simulink model "CritLike"  (R2018a)
settings: Solver=VariableStepAuto  StartTime=0.0  StopTime=0.001  RelTol=1e-3
undefined symbols (not defined in the file or in its folder): fdesignblkfcn, G1, G2, G3, G4, G5, G6, G7, G8, gcbh, get, T
libraries: dspsrcs4 x1, dspxfrm3 x1, dspobslib x1
settings Model: Creator=Daniel  LastModifiedBy=Daniel

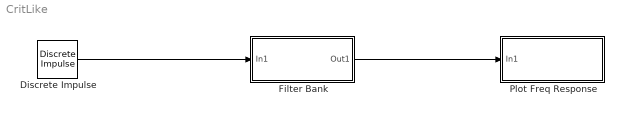
== system CritLike ==
  Discrete Impulse : dspsrcs4/Discrete  Impulse  Delay=0  SampleTime=T  FrameSample=128  OutputFrames=off  dataType=double  isSigned=on  wordLen=16  udDataType=sfix(16)  fracBitsMode=Best precision  numFracBits=15  OutDataTypeStr=double  LastOutDataTypeStr=double
  "Filter Bank " : Subsystem
  Plot Freq Response : Subsystem
  wires:
  "Filter Bank "/1(Out1) -> Plot Freq Response/1(In1)
  Discrete Impulse/1 -> "Filter Bank "/1(In1)

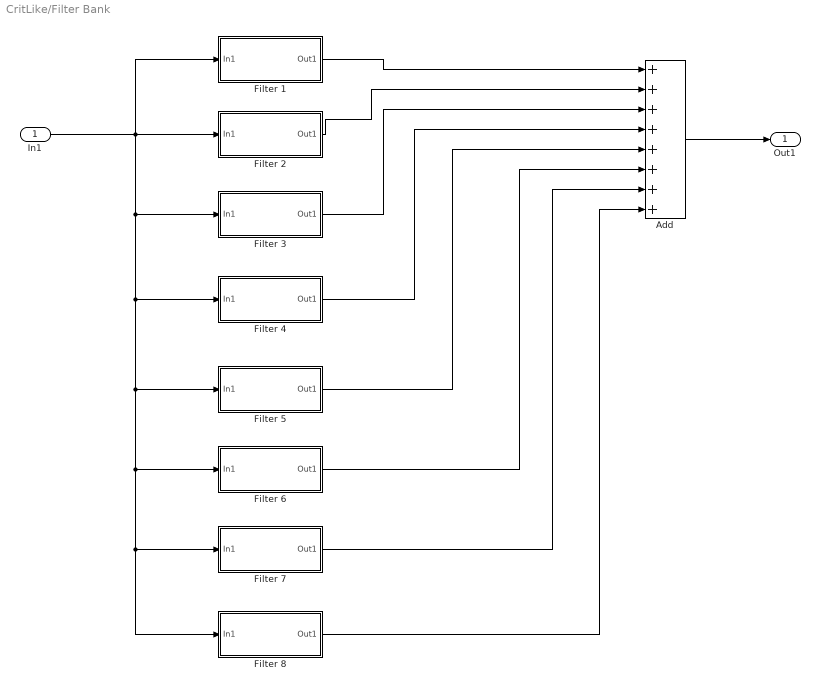
== system CritLike/Filter Bank  ==
  In1 : Inport
  Add : Sum  Inputs=++++++++
  Filter 1 : Subsystem
  Filter 2 : Subsystem
  Filter 3 : Subsystem
  Filter 4 : Subsystem
  Filter 5 : Subsystem
  Filter 6 : Subsystem
  Filter 7 : Subsystem
  Filter 8 : Subsystem
  Out1 : Outport
  wires:
  In1/1 -> Filter 3/1(In1), Filter 6/1(In1), Filter 8/1(In1), Filter 7/1(In1), Filter 5/1(In1), Filter 4/1(In1), Filter 1/1(In1), Filter 2/1(In1)
  Add/1 -> Out1/1
  Filter 1/1(Out1) -> Add/1
  Filter 2/1(Out1) -> Add/2
  Filter 3/1(Out1) -> Add/3
  Filter 4/1(Out1) -> Add/4
  Filter 5/1(Out1) -> Add/5
  Filter 6/1(Out1) -> Add/6
  Filter 7/1(Out1) -> Add/7
  Filter 8/1(Out1) -> Add/8

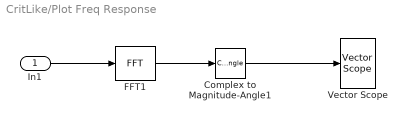
== system CritLike/Plot Freq Response ==
  In1 : Inport
  Complex to Magnitude-Angle1 : ComplexToMagnitudeAngle  Output=Magnitude
  FFT1 : dspxfrm3/FFT  FFTImplementation=Auto  CompMethod=Table lookup  TableOpt=NEW  TableOptActive=Speed  BitRevOrder=off  Normalize=off  InheritFFTLength=on  FFTLength=64  WrapInput=on  roundingMode=Floor  overflowMode=off  firstCoeffDataTypeStr=Inherit: Same word length as input  firstCoeffLastDataTypeStr=Inherit: Same word length as input  outputMin=[]  outputMax=[]
  Vector Scope : dspobslib/Vector Scope  ScopeProperties=off  Domain=Frequency  HorizSpan=1  DisplayProperties=off  AxisGrid=on  Memory=off  FrameNumber=off  AxisLegend=off  AxisZoom=off  OpenScopeAtSimStart=on  OpenScopeImmediately=off  FigPos=get(0,'defaultfigureposition')  AxisProperties=on  XUnits=Hertz  XRange=[0...Fs/2]  InheritXIncr=on  XIncr=1  XLabel=Samples  XLimit=Auto  XMin=0  XMax=1  XStart=0  YUnits=dB  YLabel=|Magnitude (dB)|  LineProperties=off  XAxisParamsVer=6.9
      settings: SourceProductName=DSP System Toolbox  SourceProductBaseCode=DS  YMin=0.0723692553519949  YMax=69.3188381671759
  wires:
  In1/1 -> FFT1/1
  FFT1/1 -> Complex to Magnitude-Angle1/1
  Complex to Magnitude-Angle1/1 -> Vector Scope/1

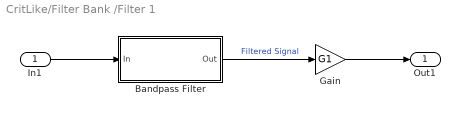
== system CritLike/Filter Bank /Filter 1 ==
  In1 : Inport
  Bandpass Filter : Subsystem  DialogController=fdesignblkfcn  InitFcn=fdesignblkfcn(gcbh, {'InitFcn'});  mask(Bandpass Filter){}
      mask help: Design a bandpass filter
      settings: CopyFcn=fdesignblkfcn(gcbh, {'CopyFcn'});
      mask Help: helpview(mapfilelocation('dsp'), 'dspbandpassfilter');
      mask Display: disp('Bandpass');
  Gain : Gain  Gain=G1
  Out1 : Outport
  wires:
  Bandpass Filter/1(Out) -> Gain/1  "Filtered Signal"
  In1/1 -> Bandpass Filter/1(In)
  Gain/1 -> Out1/1

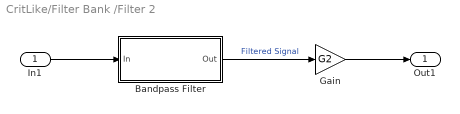
== system CritLike/Filter Bank /Filter 2 ==
  In1 : Inport
  Bandpass Filter : Subsystem  DialogController=fdesignblkfcn  InitFcn=fdesignblkfcn(gcbh, {'InitFcn'});  mask(Bandpass Filter){}
      mask help: Design a bandpass filter
      settings: CopyFcn=fdesignblkfcn(gcbh, {'CopyFcn'});
      mask Help: helpview(mapfilelocation('dsp'), 'dspbandpassfilter');
      mask Display: disp('Bandpass');
  Gain : Gain  Gain=G2
  Out1 : Outport
  wires:
  Bandpass Filter/1(Out) -> Gain/1  "Filtered Signal"
  In1/1 -> Bandpass Filter/1(In)
  Gain/1 -> Out1/1

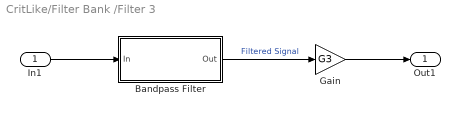
== system CritLike/Filter Bank /Filter 3 ==
  In1 : Inport
  Bandpass Filter : Subsystem  DialogController=fdesignblkfcn  InitFcn=fdesignblkfcn(gcbh, {'InitFcn'});  mask(Bandpass Filter){}
      mask help: Design a bandpass filter
      settings: CopyFcn=fdesignblkfcn(gcbh, {'CopyFcn'});
      mask Help: helpview(mapfilelocation('dsp'), 'dspbandpassfilter');
      mask Display: disp('Bandpass');
  Gain : Gain  Gain=G3
  Out1 : Outport
  wires:
  Bandpass Filter/1(Out) -> Gain/1  "Filtered Signal"
  In1/1 -> Bandpass Filter/1(In)
  Gain/1 -> Out1/1

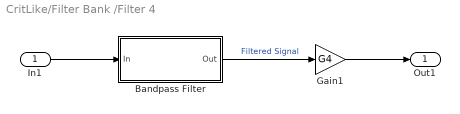
== system CritLike/Filter Bank /Filter 4 ==
  In1 : Inport
  Bandpass Filter : Subsystem  DialogController=fdesignblkfcn  InitFcn=fdesignblkfcn(gcbh, {'InitFcn'});  mask(Bandpass Filter){}
      mask help: Design a bandpass filter
      settings: CopyFcn=fdesignblkfcn(gcbh, {'CopyFcn'});
      mask Help: helpview(mapfilelocation('dsp'), 'dspbandpassfilter');
      mask Display: disp('Bandpass');
  Gain1 : Gain  Gain=G4
  Out1 : Outport
  wires:
  Bandpass Filter/1(Out) -> Gain1/1  "Filtered Signal"
  In1/1 -> Bandpass Filter/1(In)
  Gain1/1 -> Out1/1

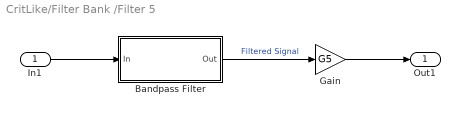
== system CritLike/Filter Bank /Filter 5 ==
  In1 : Inport
  Bandpass Filter : Subsystem  DialogController=fdesignblkfcn  InitFcn=fdesignblkfcn(gcbh, {'InitFcn'});  mask(Bandpass Filter){}
      mask help: Design a bandpass filter
      settings: CopyFcn=fdesignblkfcn(gcbh, {'CopyFcn'});
      mask Help: helpview(mapfilelocation('dsp'), 'dspbandpassfilter');
      mask Display: disp('Bandpass');
  Gain : Gain  Gain=G5
  Out1 : Outport
  wires:
  Bandpass Filter/1(Out) -> Gain/1  "Filtered Signal"
  In1/1 -> Bandpass Filter/1(In)
  Gain/1 -> Out1/1

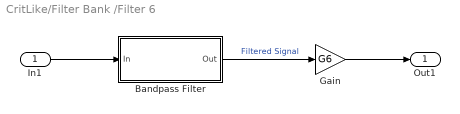
== system CritLike/Filter Bank /Filter 6 ==
  In1 : Inport
  Bandpass Filter : Subsystem  DialogController=fdesignblkfcn  InitFcn=fdesignblkfcn(gcbh, {'InitFcn'});  mask(Bandpass Filter){}
      mask help: Design a bandpass filter
      settings: CopyFcn=fdesignblkfcn(gcbh, {'CopyFcn'});
      mask Help: helpview(mapfilelocation('dsp'), 'dspbandpassfilter');
      mask Display: disp('Bandpass');
  Gain : Gain  Gain=G6
  Out1 : Outport
  wires:
  Bandpass Filter/1(Out) -> Gain/1  "Filtered Signal"
  In1/1 -> Bandpass Filter/1(In)
  Gain/1 -> Out1/1

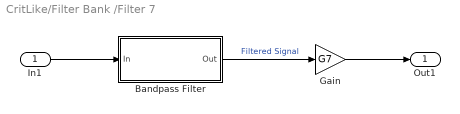
== system CritLike/Filter Bank /Filter 7 ==
  In1 : Inport
  Bandpass Filter : Subsystem  DialogController=fdesignblkfcn  InitFcn=fdesignblkfcn(gcbh, {'InitFcn'});  mask(Bandpass Filter){}
      mask help: Design a bandpass filter
      settings: CopyFcn=fdesignblkfcn(gcbh, {'CopyFcn'});
      mask Help: helpview(mapfilelocation('dsp'), 'dspbandpassfilter');
      mask Display: disp('Bandpass');
  Gain : Gain  Gain=G7
  Out1 : Outport
  wires:
  Bandpass Filter/1(Out) -> Gain/1  "Filtered Signal"
  In1/1 -> Bandpass Filter/1(In)
  Gain/1 -> Out1/1

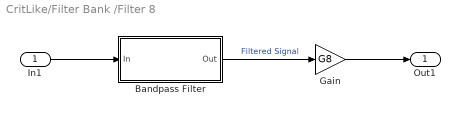
== system CritLike/Filter Bank /Filter 8 ==
  In1 : Inport
  Bandpass Filter : Subsystem  DialogController=fdesignblkfcn  InitFcn=fdesignblkfcn(gcbh, {'InitFcn'});  mask(Bandpass Filter){}
      mask help: Design a bandpass filter
      settings: CopyFcn=fdesignblkfcn(gcbh, {'CopyFcn'});
      mask Help: helpview(mapfilelocation('dsp'), 'dspbandpassfilter');
      mask Display: disp('Bandpass');
  Gain : Gain  Gain=G8
  Out1 : Outport
  wires:
  Bandpass Filter/1(Out) -> Gain/1  "Filtered Signal"
  In1/1 -> Bandpass Filter/1(In)
  Gain/1 -> Out1/1

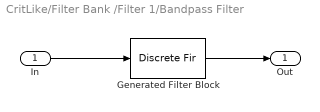
== system CritLike/Filter Bank /Filter 1/Bandpass Filter ==
  In : Inport
  Generated Filter Block : DiscreteFir  Tag=BlockMethodSubSystem  Coefficients=[0.0199963933285699849 -0.00681575804154979648 -0.00623080770076134272 -0.00599468125004754687 -0.00602772553941966979 -0.00626462816566237743 -0.00665578604798191739 -0.00716435079211600462 -0.00775634776569304393 -0.00840505905547327473 -0.00908852799300069111 -0.00978747362419878086 -0.0104811800068487851 -0.0111546244969278202 -0.0117931660813454173 -0.0123818278344493167 -0.0129056037200532721 -0.0133550366027630485 -0.013727297708585183 -0.0139618097376293 -0.0141600115498387233 -0.0141810430202207148 -0.0140822693006948108 -0.0138771537016220657 -0.0135400775563810465 -0.0130521600952322042 -0.0124170103419669643 -0.011640613742367887 -0.0107291704704825866 -0.00968587514336810909 -0.00851291407279691076 -0.00720955087776333631 -0.00578335445315706145 -0.00424624666770012649 -0.00260881143918156519 -0.00088205063409021317 0.000914112087114633126 0.00276582931342658767 0.00466895069890834596 0.00658053213214703989 0.0085153854313403457 0.0104416901824122034 0.0123364503520602929 0.0141910502600300255 0.0159892837268364174 0.0177063158886020221 0.0193255053743177606 0.0208337224473263832 0.0222161188526149508 0.0234572084633262491 0.0245474390090081006 0.0254741033555416635 0.0262236897528672214 0.0267924659178191069 0.027180389087536512 0.0273709687881046812 0.0273709687881046812 0.027180389087536512 0.0267924659178191069 0.0262236897528672214 0.0254741033555416635 0.0245474390090081006 0.0234572084633262491 0.0222161188526149508 0.0208337224473263832 0.0193255053743177606 0.0177063158886020221 0.0159892837268364174 0.0141910502600300255 0.0123364503520602929 0.0104416901824122034 0.0085153854313403457 0.00658053213214703989 0.00466895069890834596 0.00276582931342658767 0.000914112087114633126 -0.00088205063409021317 -0.00260881143918156519 -0.00424624666770012649 -0.00578335445315706145 -0.00720955087776333631 -0.00851291407279691076 -0.00968587514336810909 -0.0107291704704825866 -0.011640613742367887 -0.0124170103419669643 -0.0130521600952322042 -0.0135400775563810465 -0.0138771537016220657 -0.0140822693006948108 -0.0141810430202207148 -0.0141600115498387233 -0.0139618097376293 -0.013727297708585183 -0.0133550366027630485 -0.0129056037200532721 -0.0123818278344493167 -0.0117931660813454173 -0.0111546244969278202 -0.0104811800068487851 -0.00978747362419878086 -0.00908852799300069111 -0.00840505905547327473 -0.00775634776569304393 -0.00716435079211600462 -0.00665578604798191739 -0.00626462816566237743 -0.00602772553941966979 -0.00599468125004754687 -0.00623080770076134272 -0.00681575804154979648 0.0199963933285699849]  InputProcessing=Columns as channels (frame based)
  Out : Outport
  wires:
  In/1 -> Generated Filter Block/1
  Generated Filter Block/1 -> Out/1

== system CritLike/Filter Bank /Filter 2/Bandpass Filter ==
  In : Inport
  Generated Filter Block : DiscreteFir  Tag=BlockMethodSubSystem  Coefficients=[0.00686636152947648314 0.00291324009669534281 0.00340180636536809456 0.00384209012270262003 0.00421007194479841758 0.0044802094775745439 0.00463099935326051221 0.00464154077632829808 0.00449798169044037747 0.00418958526892799013 0.00371442857455918547 0.0030774075610790581 0.00229440500066266373 0.00138661327844640339 0.000384836897988694851 -0.000677115681057695535 -0.00175875350252952499 -0.00282007873651652719 -0.00381451527486336914 -0.00469865297808288746 -0.0054279564032785688 -0.005970978079127243 -0.00629983209626325171 -0.00640258871590675994 -0.00626496214078579514 -0.00589441195032463366 -0.00530810533648091477 -0.00455829185946255398 -0.0036604101685281205 -0.00268629826969654867 -0.0017033592629424586 -0.000768055623329439515 3.17267380095163267e-05 0.000634505432833809427 0.000964587483521655914 0.000967670265942070676 0.000589279251081043062 -0.000199344521439754203 -0.00141926008013250793 -0.00306349249454661689 -0.00511014847252137284 -0.00750915438593164394 -0.0101964547132750837 -0.0130826155874273591 -0.0160651710898091181 -0.0190224408515777994 -0.0218282792175407622 -0.0243485153570500608 -0.02645348879689308 -0.0280146990030898067 -0.028917547964700703 -0.0290636568169672545 -0.0283810672375489036 -0.0268183053710255234 -0.0243537917393071048 -0.0210008531961093439 -0.0168070744649821274 -0.0118396571017368186 -0.00621837665738500956 -6.67457583132690968e-05 0.00644909563559383382 0.013156365066465241 0.0198621811736542329 0.0263747961399391842 0.0324949614534465261 0.0380396160272325062 0.0428352384604041986 0.0467343136067170511 0.0496100217063198054 0.0513736518759769639 0.0519668317178696992 0.0513736518759769639 0.0496100217063198054 0.0467343136067170511 0.0428352384604041986 0.0380396160272325062 0.0324949614534465261 0.0263747961399391842 0.0198621811736542329 0.013156365066465241 0.00644909563559383382 -6.67457583132690968e-05 -0.00621837665738500956 -0.0118396571017368186 -0.0168070744649821274 -0.0210008531961093439 -0.0243537917393071048 -0.0268183053710255234 -0.0283810672375489036 -0.0290636568169672545 -0.028917547964700703 -0.0280146990030898067 -0.02645348879689308 -0.0243485153570500608 -0.0218282792175407622 -0.0190224408515777994 -0.0160651710898091181 -0.0130826155874273591 -0.0101964547132750837 -0.00750915438593164394 -0.00511014847252137284 -0.00306349249454661689 -0.00141926008013250793 -0.000199344521439754203 0.000589279251081043062 0.000967670265942070676 0.000964587483521655914 0.000634505432833809427 3.17267380095163267e-05 -0.000768055623329439515 -0.0017033592629424586 -0.00268629826969654867 -0.0036604101685281205 -0.00455829185946255398 -0.00530810533648091477 -0.00589441195032463366 -0.00626496214078579514 -0.00640258871590675994 -0.00629983209626325171 -0.005970978079127243 -0.0054279564032785688 -0.00469865297808288746 -0.00381451527486336914 -0.00282007873651652719 -0.00175875350252952499 -0.000677115681057695535 0.000384836897988694851 0.00138661327844640339 0.00229440500066266373 0.0030774075610790581 0.00371442857455918547 0.00418958526892799013 0.00449798169044037747 0.00464154077632829808 0.00463099935326051221 0.0044802094775745439 0.00421007194479841758 0.00384209012270262003 0.00340180636536809456 0.00291324009669534281 0.00686636152947648314]  InputProcessing=Columns as channels (frame based)
  Out : Outport
  wires:
  In/1 -> Generated Filter Block/1
  Generated Filter Block/1 -> Out/1

== system CritLike/Filter Bank /Filter 3/Bandpass Filter ==
  In : Inport
  Generated Filter Block : DiscreteFir  Tag=BlockMethodSubSystem  Coefficients=[0.00149509108830047071 -0.000642399692521037897 -0.000810630292259262265 -0.00109411713194733644 -0.00143365620682910349 -0.00177057759210485772 -0.00204842214726684048 -0.00221556181320529694 -0.00223176112355074003 -0.00207107029273874421 -0.00172840044264886347 -0.00122018591513130595 -0.000585752510254990101 0.000116848159939595344 0.000815643496512970614 0.0014337251843777243 0.00189837326751026315 0.00215174078618172787 0.00215938628032874341 0.00191755112973798791 0.00145587761015998911 0.000836765522690442526 0.00014909742389245247 -0.00050126387728264513 -0.00100513319951490033 -0.00126435563608011978 -0.00120700762496045856 -0.00079931919695550393 -5.45027824354581611e-05 0.000964615587562612435 0.00214882891085616543 0.00335180199989704641 0.00440734899131599821 0.00514602717304130704 0.00542304425625812162 0.00512672928468667962 0.00422026631943080068 0.00272086574312288337 0.000722652626853492459 -0.00160768236526998291 -0.00405692337631967555 -0.00637979596434344858 -0.00833229639845109969 -0.00969480631771980038 -0.0103066726647600398 -0.0100832788511609449 -0.00903380550389796047 -0.00726066016671503712 -0.00495321220269955616 -0.00236449281411958831 0.000216473219440355737 0.00250309087081964548 0.00424656717563655275 0.00527285211275412783 0.00550669870442097378 0.00498857474890576722 0.00387194054481450811 0.00240999857559025862 0.000922884027534769395 -0.000241586805852883813 -0.000759012989260025015 -0.000375259651860081287 0.00104719868262927217 0.00349944902901677679 0.00680854713042963917 0.0106442340573191779 0.0145433659020440722 0.0179559352420405327 0.0203056745893020231 0.021058775959816832 0.0197971035980004303 0.0162778767692930079 0.0104845628866556389 0.00265586520359594336 -0.00672305424159115855 -0.0169424913846908491 -0.0271298514931554054 -0.0363229150875501172 -0.0435707911460218381 -0.0480268436849823066 -0.0490459506983308771 -0.0462609439436757058 -0.0396372026139303474 -0.0294927332204201892 -0.0164860529732185936 -0.00156580171800659138 0.0141070284234607619 0.0292646785419930291 0.0426468672267536625 0.0531218125877600186 0.0597915487149781946 0.0620811305353086776 0.0597915487149781946 0.0531218125877600186 0.0426468672267536625 0.0292646785419930291 0.0141070284234607619 -0.00156580171800659138 -0.0164860529732185936 -0.0294927332204201892 -0.0396372026139303474 -0.0462609439436757058 -0.0490459506983308771 -0.0480268436849823066 -0.0435707911460218381 -0.0363229150875501172 -0.0271298514931554054 -0.0169424913846908491 -0.00672305424159115855 0.00265586520359594336 0.0104845628866556389 0.0162778767692930079 0.0197971035980004303 0.021058775959816832 0.0203056745893020231 0.0179559352420405327 0.0145433659020440722 0.0106442340573191779 0.00680854713042963917 0.00349944902901677679 0.00104719868262927217 -0.000375259651860081287 -0.000759012989260025015 -0.000241586805852883813 0.000922884027534769395 0.00240999857559025862 0.00387194054481450811 0.00498857474890576722 0.00550669870442097378 0.00527285211275412783 0.00424656717563655275 0.00250309087081964548 0.000216473219440355737 -0.00236449281411958831 -0.00495321220269955616 -0.00726066016671503712 -0.00903380550389796047 -0.0100832788511609449 -0.0103066726647600398 -0.00969480631771980038 -0.00833229639845109969 -0.00637979596434344858 -0.00405692337631967555 -0.00160768236526998291 0.000722652626853492459 0.00272086574312288337 0.00422026631943080068 0.00512672928468667962 0.00542304425625812162 0.00514602717304130704 0.00440734899131599821 0.00335180199989704641 0.00214882891085616543 0.000964615587562612435 -5.45027824354581611e-05 -0.00079931919695550393 -0.00120700762496045856 -0.00126435563608011978 -0.00100513319951490033 -0.00050126387728264513 0.00014909742389245247 0.000836765522690442526 0.00145587761015998911 0.00191755112973798791 0.00215938628032874341 0.00215174078618172787 0.00189837326751026315 0.0014337251843777243 0.000815643496512970614 0.000116848159939595344 -0.000585752510254990101 -0.00122018591513130595 -0.00172840044264886347 -0.00207107029273874421 -0.00223176112355074003 -0.00221556181320529694 -0.00204842214726684048 -0.00177057759210485772 -0.00143365620682910349 -0.00109411713194733644 -0.000810630292259262265 -0.000642399692521037897 0.00149509108830047071]  InputProcessing=Columns as channels (frame based)
  Out : Outport
  wires:
  In/1 -> Generated Filter Block/1
  Generated Filter Block/1 -> Out/1

== system CritLike/Filter Bank /Filter 4/Bandpass Filter ==
  In : Inport
  Generated Filter Block : DiscreteFir  Tag=BlockMethodSubSystem  Coefficients=[-0.00150190139865964993 0.000488356422976355775 0.000631973387870471393 0.000832516372821275855 0.00101201257816564021 0.00109790155191552856 0.00103717026429450796 0.000809024479108051611 0.000431037136996139855 -4.15198941371832731e-05 -0.000526743967803182194 -0.000933310808923894794 -0.00118144104044380074 -0.0012226104038448901 -0.00105276718868126313 -0.000714921541033167358 -0.000290264610615555499 0.000121126808649581275 0.000425598012469503579 0.000560983971146497454 0.000514822684227278851 0.000330314500978377335 9.73032325550369137e-05 -7.09794289107746397e-05 -7.00667969772721442e-05 0.000161703164242938497 0.000616896954026145542 0.00120874561728147095 0.00178185800977157297 0.00214248603133814939 0.00210658416334724014 0.00155091723697160441 0.000458093017498411431 -0.00105963607154432068 -0.00276053463033785118 -0.00432232287568423169 -0.00537437427840396949 -0.0056097187343710931 -0.00484282978257280592 -0.00307141570578481132 -0.000501083872473292004 0.0024745299158579221 0.00533766971369815848 0.0075423128674817104 0.00862559947417160938 0.0083094571652135487 0.00657026960705265305 0.00365889363524963141 6.32739912582283885e-05 -0.00358167098670209884 -0.00661931905040888478 -0.00850604615805119167 -0.00892581141013616859 -0.00785806433778807149 -0.00558206009896857012 -0.00261454981810105291 0.000406931480766468869 0.0028701951695335663 0.00432986462451839024 0.00461141843131849822 0.00385074172212267109 0.00245692416909795664 0.00100415311652434381 7.82137320039329371e-05 0.000108028642745487289 0.00123142692050522617 0.00322565288974955905 0.00552951902618499004 0.00735631906035747601 0.00788427280031177985 0.00646952917146487259 0.00285826889124905564 -0.00268531698152329199 -0.00935372548077310212 -0.0158990373126559059 -0.0208542400402678581 -0.0228350322464138458 -0.0208610025930315579 -0.0146280289652055973 -0.00466517625401003614 0.00766896347069463257 0.0203654686995357707 0.0310983200176112203 0.0376556167035752148 0.0383872416090329308 0.0325786289594396442 0.0206692229451644824 0.0042604486658585879 -0.0141021190730410886 -0.0313429093577956078 -0.0443964075176603301 -0.0507747850606430004 -0.0490533260004177019 -0.0391779185273584893 -0.022527962963586997 -0.00171450986509646118 0.0198555711717661142 0.0385691763764611159 0.0512521088812927517 0.0557360815320822947 0.0512521088812927517 0.0385691763764611159 0.0198555711717661142 -0.00171450986509646118 -0.022527962963586997 -0.0391779185273584893 -0.0490533260004177019 -0.0507747850606430004 -0.0443964075176603301 -0.0313429093577956078 -0.0141021190730410886 0.0042604486658585879 0.0206692229451644824 0.0325786289594396442 0.0383872416090329308 0.0376556167035752148 0.0310983200176112203 0.0203654686995357707 0.00766896347069463257 -0.00466517625401003614 -0.0146280289652055973 -0.0208610025930315579 -0.0228350322464138458 -0.0208542400402678581 -0.0158990373126559059 -0.00935372548077310212 -0.00268531698152329199 0.00285826889124905564 0.00646952917146487259 0.00788427280031177985 0.00735631906035747601 0.00552951902618499004 0.00322565288974955905 0.00123142692050522617 0.000108028642745487289 7.82137320039329371e-05 0.00100415311652434381 0.00245692416909795664 0.00385074172212267109 0.00461141843131849822 0.00432986462451839024 0.0028701951695335663 0.000406931480766468869 -0.00261454981810105291 -0.00558206009896857012 -0.00785806433778807149 -0.00892581141013616859 -0.00850604615805119167 -0.00661931905040888478 -0.00358167098670209884 6.32739912582283885e-05 0.00365889363524963141 0.00657026960705265305 0.0083094571652135487 0.00862559947417160938 0.0075423128674817104 0.00533766971369815848 0.0024745299158579221 -0.000501083872473292004 -0.00307141570578481132 -0.00484282978257280592 -0.0056097187343710931 -0.00537437427840396949 -0.00432232287568423169 -0.00276053463033785118 -0.00105963607154432068 0.000458093017498411431 0.00155091723697160441 0.00210658416334724014 0.00214248603133814939 0.00178185800977157297 ...(+674 chars)]  InputProcessing=Columns as channels (frame based)
  Out : Outport
  wires:
  In/1 -> Generated Filter Block/1
  Generated Filter Block/1 -> Out/1

== system CritLike/Filter Bank /Filter 5/Bandpass Filter ==
  In : Inport
  Generated Filter Block : DiscreteFir  Tag=BlockMethodSubSystem  Coefficients=[0.0021986710633923102 -0.000123703446631435142 -0.000696905120939670872 -0.0014253796291338796 -0.0020042974150217361 -0.00212531777926342836 -0.00160170442605077606 -0.000460601928675574094 0.00102465615146940785 0.00240410312400101724 0.00319116347169363587 0.00304514595799531499 0.00190619875140471732 5.26685322279956888e-05 -0.00197352168257558004 -0.00351784028346037361 -0.00407345140038681795 -0.00343332340617129653 -0.00178692833087177867 0.000337865086840349275 0.00226998095411966132 0.00342447156003534373 0.00351613685735909778 0.0026415554754949588 0.00122193770249327447 -0.000189098440497991339 -0.00113304255974914841 -0.001430988109810169 -0.0012308462819895546 -0.000911119222355132518 -0.00085928034224075139 -0.00125626263065418704 -0.00194397614818719259 -0.00245982168403965527 -0.00224441272554694402 -0.000926767887369655185 0.00142026376457112143 0.00419604356849941941 0.00641526584891172029 0.00705614810713682018 0.00548606476309891622 0.00179742317186433248 -0.0031033609035481689 -0.00772082981105184484 -0.0104613876587561667 -0.0102146890292074792 -0.00681017027183695133 -0.00115955645442004972 0.0050050037810786584 0.00970912131840214951 0.0114420149114788788 0.00971045059010767521 0.00522705223621743043 -0.000358947965815038707 -0.00509319792272372885 -0.00747088085691407448 -0.00701138801436937929 -0.00441442771891371009 -0.00121878538558460679 0.000903378876412276773 0.000928366217242118305 -0.000999931468447917086 -0.00356817491343113359 -0.00484284054692180228 -0.00318419566479350748 0.00185520056615331693 0.00905146669080701335 0.0157200056617022403 0.0186241932598827445 0.0152899680681256745 0.0052323926055284041 -0.00943233662417152993 -0.0243273278995200723 -0.034108531150648401 -0.0343315737095081924 -0.0232499845602912383 -0.00284596648016663834 0.0213735630351935268 0.041884977657597855 0.0515382353356195685 0.0460556597764364278 0.0257599495504530172 -0.00414241204038749526 -0.0349241960332123888 -0.0569871908762738591 -0.0629627705378366098 -0.0502311399772133599 -0.021978751176083125 0.0136172364956398569 0.0458675002631019901 0.0649249082206462269 0.0649249082206462269 0.0458675002631019901 0.0136172364956398569 -0.021978751176083125 -0.0502311399772133599 -0.0629627705378366098 -0.0569871908762738591 -0.0349241960332123888 -0.00414241204038749526 0.0257599495504530172 0.0460556597764364278 0.0515382353356195685 0.041884977657597855 0.0213735630351935268 -0.00284596648016663834 -0.0232499845602912383 -0.0343315737095081924 -0.034108531150648401 -0.0243273278995200723 -0.00943233662417152993 0.0052323926055284041 0.0152899680681256745 0.0186241932598827445 0.0157200056617022403 0.00905146669080701335 0.00185520056615331693 -0.00318419566479350748 -0.00484284054692180228 -0.00356817491343113359 -0.000999931468447917086 0.000928366217242118305 0.000903378876412276773 -0.00121878538558460679 -0.00441442771891371009 -0.00701138801436937929 -0.00747088085691407448 -0.00509319792272372885 -0.000358947965815038707 0.00522705223621743043 0.00971045059010767521 0.0114420149114788788 0.00970912131840214951 0.0050050037810786584 -0.00115955645442004972 -0.00681017027183695133 -0.0102146890292074792 -0.0104613876587561667 -0.00772082981105184484 -0.0031033609035481689 0.00179742317186433248 0.00548606476309891622 0.00705614810713682018 0.00641526584891172029 0.00419604356849941941 0.00142026376457112143 -0.000926767887369655185 -0.00224441272554694402 -0.00245982168403965527 -0.00194397614818719259 -0.00125626263065418704 -0.00085928034224075139 -0.000911119222355132518 -0.0012308462819895546 -0.001430988109810169 -0.00113304255974914841 -0.000189098440497991339 0.00122193770249327447 0.0026415554754949588 0.00351613685735909778 0.00342447156003534373 0.00226998095411966132 0.000337865086840349275 -0.00178692833087177867 -0.00343332340617129653 -0.00407345140038681795 -0.00351784028346037361 -0.00197352168257558004 5.26685322279956888e-05 0.00190619875140471732 0.00304514595799531499 0.00319116347169363587 0.00240410312400101724 0.00102465615146940785 -0.000460601928675574094 -0.00160170442605077606 -0.00212531777926342836 -0.0020042974150217361 -0.0014253796291338796 -0.000696905120939670872 -0.000123703446631435142 0.0021986710633923102]  InputProcessing=Columns as channels (frame based)
  Out : Outport
  wires:
  In/1 -> Generated Filter Block/1
  Generated Filter Block/1 -> Out/1

== system CritLike/Filter Bank /Filter 6/Bandpass Filter ==
  In : Inport
  Generated Filter Block : DiscreteFir  Tag=BlockMethodSubSystem  Coefficients=[0.00264579793748627619 -0.000102407615892199827 -0.00095886888172079369 -0.00179718476565946428 -0.00201497960296586264 -0.00133494893499796 -2.36741214705326721e-05 0.00123137358862371554 0.00174436766169009435 0.00126999624799908526 0.00016157698393464589 -0.000881177639932187017 -0.00129447440733165787 -0.00102412258528767328 -0.00050320512538661532 -0.00025449138225583682 -0.000416291901857523993 -0.00059167622197051138 -0.000174916436453063663 0.00104836164492139216 0.00251499435315213687 0.00308744722458186059 0.00183298227968287748 -0.00113747873233549512 -0.00441140223198479599 -0.00594501435773542655 -0.00433615151898993773 8.01126265023841997e-05 0.00513688998166454344 0.0079411532910977408 0.00664086904546424932 0.00167456682785334095 -0.00433427096104945127 -0.00804575309593332649 -0.00744774333922400625 -0.00305977254721840697 0.00241466504281432704 0.00584962816237051108 0.00565853528688943248 0.00267979684507604074 -0.000623752578715030528 -0.0020314098609961178 -0.00116369598543100239 0.00037885337268020084 0.000430618481325302168 -0.00180960452538885073 -0.00485433800460873845 -0.00582509478337783076 -0.00267631688155832177 0.00386385074133913315 0.0101833654312149472 0.0118775711356551451 0.00677982316038782187 -0.00313909518081499032 -0.012515886605688099 -0.0157370328351381025 -0.0105510702407515342 0.00030055298455617833 0.0106426300998888057 0.0147248134563475307 0.0108298830640973977 0.00220821735670513218 -0.0053594675375063577 -0.00764766606236797885 -0.0048265502913504817 -0.000962684666750616524 -0.000490290971639982987 -0.00427823384977308024 -0.00840414949885705427 -0.00693772347633384284 0.00297683749778708756 0.0174864530674708855 0.0270524727887331146 0.0222976325311557526 0.00122989433339355868 -0.0272398548971825062 -0.0467739593922700328 -0.0429650591528363338 -0.0132008570169620549 0.0294933360699324958 0.062065851246150279 0.0641819254958263113 0.0308974866952659473 -0.0226661137271557921 -0.0683072223229584663 -0.0801209518882364247 -0.0496105623946079197 0.00849265640873767338 0.0636070994254838706 0.0860406426715831646 0.0636070994254838706 0.00849265640873767338 -0.0496105623946079197 -0.0801209518882364247 -0.0683072223229584663 -0.0226661137271557921 0.0308974866952659473 0.0641819254958263113 0.062065851246150279 0.0294933360699324958 -0.0132008570169620549 -0.0429650591528363338 -0.0467739593922700328 -0.0272398548971825062 0.00122989433339355868 0.0222976325311557526 0.0270524727887331146 0.0174864530674708855 0.00297683749778708756 -0.00693772347633384284 -0.00840414949885705427 -0.00427823384977308024 -0.000490290971639982987 -0.000962684666750616524 -0.0048265502913504817 -0.00764766606236797885 -0.0053594675375063577 0.00220821735670513218 0.0108298830640973977 0.0147248134563475307 0.0106426300998888057 0.00030055298455617833 -0.0105510702407515342 -0.0157370328351381025 -0.012515886605688099 -0.00313909518081499032 0.00677982316038782187 0.0118775711356551451 0.0101833654312149472 0.00386385074133913315 -0.00267631688155832177 -0.00582509478337783076 -0.00485433800460873845 -0.00180960452538885073 0.000430618481325302168 0.00037885337268020084 -0.00116369598543100239 -0.0020314098609961178 -0.000623752578715030528 0.00267979684507604074 0.00565853528688943248 0.00584962816237051108 0.00241466504281432704 -0.00305977254721840697 -0.00744774333922400625 -0.00804575309593332649 -0.00433427096104945127 0.00167456682785334095 0.00664086904546424932 0.0079411532910977408 0.00513688998166454344 8.01126265023841997e-05 -0.00433615151898993773 -0.00594501435773542655 -0.00441140223198479599 -0.00113747873233549512 0.00183298227968287748 0.00308744722458186059 0.00251499435315213687 0.00104836164492139216 -0.000174916436453063663 -0.00059167622197051138 -0.000416291901857523993 -0.00025449138225583682 -0.00050320512538661532 -0.00102412258528767328 -0.00129447440733165787 -0.000881177639932187017 0.00016157698393464589 0.00126999624799908526 0.00174436766169009435 0.00123137358862371554 -2.36741214705326721e-05 -0.00133494893499796 -0.00201497960296586264 -0.00179718476565946428 -0.00095886888172079369 -0.000102407615892199827 0.00264579793748627619]  InputProcessing=Columns as channels (frame based)
  Out : Outport
  wires:
  In/1 -> Generated Filter Block/1
  Generated Filter Block/1 -> Out/1

== system CritLike/Filter Bank /Filter 7/Bandpass Filter ==
  In : Inport
  Generated Filter Block : DiscreteFir  Tag=BlockMethodSubSystem  Coefficients=[-0.00242620292658780228 0.000781087018450470397 0.00127816581772777064 0.000938695163573566283 0.000614128685171459092 0.00125468376048931403 0.00140212779049935584 -0.000930643773456046918 -0.00386997881201199849 -0.00264738578145360705 0.00326626417172270469 0.00721016275927415917 0.00318593996688394535 -0.00509720912241106924 -0.00780934776429196599 -0.00181516879936189659 0.00510815581786191065 0.00504951206831110236 0.000241072642053247671 -0.00181253457285809579 -1.67678191570371142e-05 5.01152498152696775e-05 -0.00320658541264187561 -0.00393198754013688017 0.00128430021264623411 0.00643351493306067775 0.00435136187541197011 -0.00224840014106832131 -0.00475981212488886269 -0.00161512407201707384 0.000489629688932233633 -0.00132154260937504542 -0.00129035065741198293 0.00396781203950785123 0.00743366712547030573 0.00175927036080061666 -0.00757782788063389445 -0.00855736687159950118 -0.000242683223833181123 0.00586789200057558167 0.00344235819931185865 -0.000164077115036157162 0.00202997379078577542 0.00393683989196669335 -0.00262873723002628613 -0.0111317342745260398 -0.00768380608249157569 0.00641250266762940883 0.0136650714918644389 0.00537624977716551905 -0.00572747784967772653 -0.00573881976175451367 -0.000389581219181391958 -0.00262782834143748855 -0.00813378895234547969 -0.00158514947451503631 0.014452250209581451 0.0175220500381466256 -0.00107229921899071692 -0.0192362263753971356 -0.0144986252326571793 0.00316369662942122491 0.00846327435986695721 0.000997085356944710103 0.00250348668371602788 0.0150142513243875994 0.0120410618237255899 -0.0159798337900946066 -0.0353658137615115373 -0.014137749319292613 0.0253472735827468335 0.0334211063513671566 0.00564645571415699817 -0.0126611139953301342 -0.00147725408002078395 0.000642122159866198691 -0.0318870046242088409 -0.0484619428304257915 0.0105111768649120991 0.0984100887566332211 0.0907498853920805787 -0.0426609739946615385 -0.158982302577681089 -0.103034139163780139 0.081499496150434711 0.183481489219564697 0.081499496150434711 -0.103034139163780139 -0.158982302577681089 -0.0426609739946615385 0.0907498853920805787 0.0984100887566332211 0.0105111768649120991 -0.0484619428304257915 -0.0318870046242088409 0.000642122159866198691 -0.00147725408002078395 -0.0126611139953301342 0.00564645571415699817 0.0334211063513671566 0.0253472735827468335 -0.014137749319292613 -0.0353658137615115373 -0.0159798337900946066 0.0120410618237255899 0.0150142513243875994 0.00250348668371602788 0.000997085356944710103 0.00846327435986695721 0.00316369662942122491 -0.0144986252326571793 -0.0192362263753971356 -0.00107229921899071692 0.0175220500381466256 0.014452250209581451 -0.00158514947451503631 -0.00813378895234547969 -0.00262782834143748855 -0.000389581219181391958 -0.00573881976175451367 -0.00572747784967772653 0.00537624977716551905 0.0136650714918644389 0.00641250266762940883 -0.00768380608249157569 -0.0111317342745260398 -0.00262873723002628613 0.00393683989196669335 0.00202997379078577542 -0.000164077115036157162 0.00344235819931185865 0.00586789200057558167 -0.000242683223833181123 -0.00855736687159950118 -0.00757782788063389445 0.00175927036080061666 0.00743366712547030573 0.00396781203950785123 -0.00129035065741198293 -0.00132154260937504542 0.000489629688932233633 -0.00161512407201707384 -0.00475981212488886269 -0.00224840014106832131 0.00435136187541197011 0.00643351493306067775 0.00128430021264623411 -0.00393198754013688017 -0.00320658541264187561 5.01152498152696775e-05 -1.67678191570371142e-05 -0.00181253457285809579 0.000241072642053247671 0.00504951206831110236 0.00510815581786191065 -0.00181516879936189659 -0.00780934776429196599 -0.00509720912241106924 0.00318593996688394535 0.00721016275927415917 0.00326626417172270469 -0.00264738578145360705 -0.00386997881201199849 -0.000930643773456046918 0.00140212779049935584 0.00125468376048931403 0.000614128685171459092 0.000938695163573566283 0.00127816581772777064 0.000781087018450470397 -0.00242620292658780228]  InputProcessing=Columns as channels (frame based)
  Out : Outport
  wires:
  In/1 -> Generated Filter Block/1
  Generated Filter Block/1 -> Out/1

== system CritLike/Filter Bank /Filter 8/Bandpass Filter ==
  In : Inport
  Generated Filter Block : DiscreteFir  Tag=BlockMethodSubSystem  Coefficients=[-0.00094183346819342944 -0.0106688451512830379 0.0187556807071922321 -0.0108515944433483745 -0.00293052956451312491 0.00361122443932587744 0.00155962220211500885 0.00234606927751747352 -0.00646706074635001321 0.000767785875835435422 0.00335490501608611338 -0.000389963750683376686 0.00179121789112192745 -0.00632429692035619065 0.00242578845671614224 0.00334605737535930564 -0.00137760400180047399 0.00119240074436185312 -0.00644720556895141822 0.00432977019750778458 0.00314608159786009325 -0.00258433815047521762 0.000607031650950499296 -0.00616581722659715822 0.00650513310145069829 0.00232770659689521264 -0.00412534401529863343 0.000394603413364010003 -0.0053086559405361132 0.00868348181915023012 0.000593871457877748893 -0.00578924462528453837 0.000901576109682528104 -0.00393247872018617425 0.0104814792191614894 -0.00218337434309327783 -0.00719203218545799022 0.00239817882979274227 -0.00231286451142924399 0.0115328969019290739 -0.00597800537817149563 -0.00782822620056094348 0.00502217992794623536 -0.000905682918942881526 0.0115369426260608053 -0.010587039928964391 -0.00713066842145507196 0.00874520887803339336 -0.00033145302875241256 0.010337418134551038 -0.0156673315060838689 -0.00449254297095441103 0.0133455934813170429 -0.00136922417889739564 0.00800377657592019412 -0.020799840607944528 0.000739852687187556035 0.0184412979397590784 -0.00503290037985235084 0.00491286503530652743 -0.0256388025196309724 0.00950184682598981777 0.0234976233519120607 -0.0128315213204651946 0.00178204308583594304 -0.030114246826308963 0.0238198026043740033 0.0279428249026747455 -0.0282409401922187019 0.000123159942935352484 -0.0351817522241806846 0.0507045879631156521 0.0312667959390658806 -0.0650621029510657506 0.00530343676564722089 -0.0478561455670731897 0.139075460336841261 0.0330351425530121534 -0.321501820603640964 0.211636974631660646 0.211636974631660646 -0.321501820603640964 0.0330351425530121534 0.139075460336841261 -0.0478561455670731897 0.00530343676564722089 -0.0650621029510657506 0.0312667959390658806 0.0507045879631156521 -0.0351817522241806846 0.000123159942935352484 -0.0282409401922187019 0.0279428249026747455 0.0238198026043740033 -0.030114246826308963 0.00178204308583594304 -0.0128315213204651946 0.0234976233519120607 0.00950184682598981777 -0.0256388025196309724 0.00491286503530652743 -0.00503290037985235084 0.0184412979397590784 0.000739852687187556035 -0.020799840607944528 0.00800377657592019412 -0.00136922417889739564 0.0133455934813170429 -0.00449254297095441103 -0.0156673315060838689 0.010337418134551038 -0.00033145302875241256 0.00874520887803339336 -0.00713066842145507196 -0.010587039928964391 0.0115369426260608053 -0.000905682918942881526 0.00502217992794623536 -0.00782822620056094348 -0.00597800537817149563 0.0115328969019290739 -0.00231286451142924399 0.00239817882979274227 -0.00719203218545799022 -0.00218337434309327783 0.0104814792191614894 -0.00393247872018617425 0.000901576109682528104 -0.00578924462528453837 0.000593871457877748893 0.00868348181915023012 -0.0053086559405361132 0.000394603413364010003 -0.00412534401529863343 0.00232770659689521264 0.00650513310145069829 -0.00616581722659715822 0.000607031650950499296 -0.00258433815047521762 0.00314608159786009325 0.00432977019750778458 -0.00644720556895141822 0.00119240074436185312 -0.00137760400180047399 0.00334605737535930564 0.00242578845671614224 -0.00632429692035619065 0.00179121789112192745 -0.000389963750683376686 0.00335490501608611338 0.000767785875835435422 -0.00646706074635001321 0.00234606927751747352 0.00155962220211500885 0.00361122443932587744 -0.00293052956451312491 -0.0108515944433483745 0.0187556807071922321 -0.0106688451512830379 -0.00094183346819342944]  InputProcessing=Columns as channels (frame based)
  Out : Outport
  wires:
  In/1 -> Generated Filter Block/1
  Generated Filter Block/1 -> Out/1
